simulink model "ModelHeatTreatment_FMU"  (R2020b)
settings: Solver=FixedStepAuto  StartTime=0.0  StopTime=Inf  FixedStep=0.010  RelTol=1e-3
settings Model: Creator=kaebi  LastModifiedBy=kaebi
settings OptimizationCC: DefaultParameterBehavior=Inlined  LocalBlockOutputs=off
settings RTWCC: GenCodeOnly=on

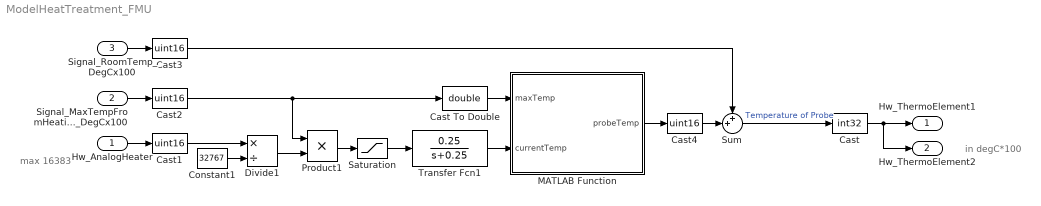
== system ModelHeatTreatment_FMU ==
  note: max 16383
  note: in degC*100
  Hw_AnalogHeater : Inport  OutDataTypeStr=int32
  Signal_MaxTempFromHeating_DegCx100 : Inport  Port=2  OutDataTypeStr=int32
  Signal_RoomTemp_DegCx100 : Inport  Port=3  OutDataTypeStr=int32
  Cast : DataTypeConversion  OutDataTypeStr=int32
  Cast To Double : DataTypeConversion  OutDataTypeStr=double
  Cast{1..4} (4 alike) : DataTypeConversion  OutDataTypeStr=uint16
  Constant1 : Constant  Value=32767
  Divide1 : Product  Inputs=*/  OutDataTypeStr=double
  MATLAB Function : MATLAB Function  TreatAsAtomicUnit=on
  Product1 : Product
  Saturation : Saturate  UpperLimit=inf  LowerLimit=0
  Sum : Sum  Inputs=++|
  Transfer Fcn1 : TransferFcn  Numerator=[0.25]  Denominator=[1 0.25]
  Hw_ThermoElement1 : Outport  OutDataTypeStr=int32
  Hw_ThermoElement2 : Outport  Port=2  OutDataTypeStr=int32
  wires:
  Signal_RoomTemp_DegCx100/1 -> Cast3/1
  Sum/1 -> Cast/1  "Temperature of Probe"
  MATLAB Function/1(probeTemp) -> Cast4/1
  Constant1/1 -> Divide1/2
  Divide1/1 -> Product1/2
  Product1/1 -> Saturation/1
  Transfer Fcn1/1 -> MATLAB Function/2(currentTemp)
  Hw_AnalogHeater/1 -> Cast1/1
  Saturation/1 -> Transfer Fcn1/1
  Signal_MaxTempFromHeating_DegCx100/1 -> Cast2/1
  Cast To Double/1 -> MATLAB Function/1(maxTemp)
  Cast1/1 -> Divide1/1
  Cast2/1 -> Product1/1, Cast To Double/1
  Cast3/1 -> Sum/1
  Cast4/1 -> Sum/2
  Cast/1 -> Hw_ThermoElement2/1, Hw_ThermoElement1/1

== matlab function ModelHeatTreatment_FMU/MATLAB Function ==
  data: maxTemp input; probeTemp output; currentTemp input
function probeTemp = TemperatureModel(maxTemp, currentTemp)

if (currentTemp < 0)
    currentTemp = 0;
elseif (currentTemp > maxTemp)
    currentTemp = maxTemp;
end


probeTemp = currentTemp;
